simulink model "LimKyuBum_20101447_6_continuous"  (R2017a)
settings: Solver=ode4  StartTime=0.0  StopTime=10.0  FixedStep=0.01  RelTol=1e-3
model workspace (MAT data in the model file):
  K = 1000
  U = 10000
  b = 50
  m = 1000
settings Model: Creator=508-104  LastModifiedBy=508-104
settings DebuggingCC: MaxConsecutiveZCsMsg=none

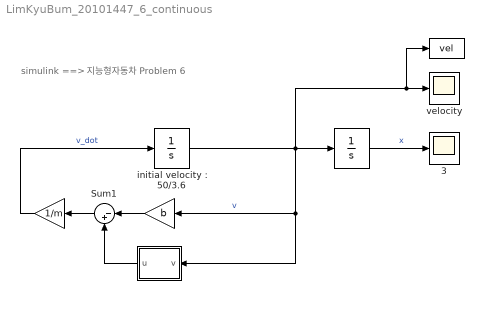
== system LimKyuBum_20101447_6_continuous ==
  note: simulink ==> 지능형자동차 Problem 6
  " " : Gain  Gain=b
  "  " : Subsystem
  "    " : Gain  Gain=1/m
  "     " : ToWorkspace  VariableName=vel  SaveFormat=Timeseries  SampleTime=-1
  "      " : Integrator
  " 3" : Scope
  " velocity" : Scope
  Sum1 : Sum  Inputs=|-+
  "initial velocity : 50/3.6" : Integrator  InitialCondition=50/3.6
  wires:
  "initial velocity : 50/3.6"/1 -> "      "/1, "  "/1(v), " "/1, "     "/1, " velocity"/1  "v"
  "    "/1 -> "initial velocity : 50/3.6"/1  "v_dot"
  " "/1 -> Sum1/1
  "  "/1(u) -> Sum1/2
  Sum1/1 -> "    "/1
  "      "/1 -> " 3"/1  "x"

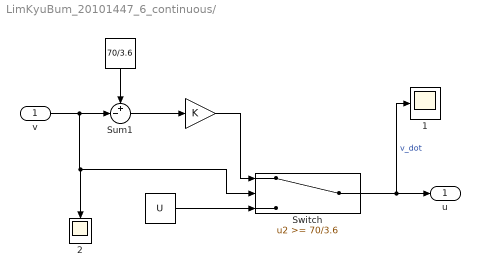
== system LimKyuBum_20101447_6_continuous/   ==
  v : Inport
  " " : Constant  Value=70/3.6
  "  " : Gain  Gain=K
  "    " : Constant  Value=U
  " 1" : Scope
  " 2" : Scope
  Sum1 : Sum  Inputs=+-|
  Switch : Switch  Threshold=70/3.6
  u : Outport
  wires:
  "  "/1 -> Switch/1
  " "/1 -> Sum1/1
  "    "/1 -> Switch/3
  Switch/1 -> " 1"/1, u/1  "v_dot"
  v/1 -> Switch/2, " 2"/1, Sum1/2
  Sum1/1 -> "  "/1
